simulink model "ysw_PID2"  (Simulink 8.3)
settings: Solver=ode45  StartTime=0.0  StopTime=10  RelTol=1e-3
values from neighbouring files (symbols this model uses):
  A = [  0 ,     1,                 0                 0 ... (first row only)    [ysw_PID.m]
  B = [0;  (I+m*l^2)/((M+m)*I+M*m*l^2);  0;  m*l/(((M+m)*I+M*m*l^2))]    [ysw_PID.m]
  C = [1 0 0 0;0 1 0 0;0 0 1 0;0 0 0 1]    [ysw_PID.m]
  D = [0;0;0;0]    [ysw_PID.m]
  K = place(A,B,p)    [ysw_PID.m]
libraries: simulink x1
settings Model: Creator=ii  LastModifiedBy=ii
settings SolverCC: ZeroCrossAlgorithm=Adaptive
settings DataIOCC: SignalLoggingSaveFormat=Dataset
settings DebuggingCC: StateNameClashWarn=none
settings GRTTargetCC: CombineOutputUpdateFcns=on  GRTInterface=off

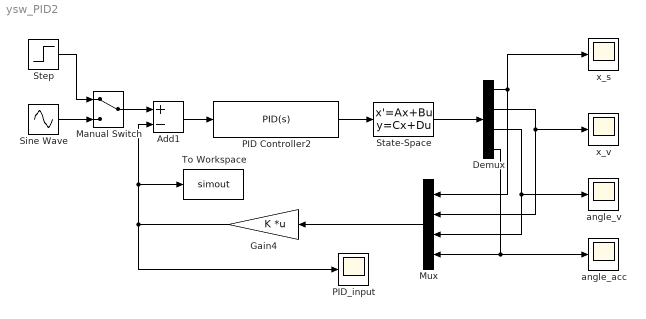
== system ysw_PID2 ==
  Add1 : Sum  Inputs=+-
  Demux : Demux
  Gain4 : Gain  Gain=K  Multiplication=Matrix(K*u)
  Manual Switch : ManualSwitch
  Mux : Mux
  PID Controller2 : simulink/Continuous/PID Controller  Controller=PID  TimeDomain=Continuous-time  SampleTime=1  IntegratorMethod=Forward Euler  FilterMethod=Forward Euler  Form=Parallel  P=5  I=0.001  D=1  N=100  InitialConditionSource=internal  InitialConditionForIntegrator=0  InitialConditionForFilter=0  ExternalReset=none  LimitOutput=off  UpperSaturationLimit=inf  LowerSaturationLimit=-inf  LinearizeAsGain=on  AntiWindupMode=none  Kb=1  TrackingMode=off  Kt=1  PParamMin=[]  PParamMax=[]  IParamMin=[]  IParamMax=[]  DParamMin=[]  DParamMax=[]  NParamMin=[]  NParamMax=[]  KbParamMin=[]  KbParamMax=[]  KtParamMin=[]  KtParamMax=[]  POutMin=[]  POutMax=[]  IOutMin=[]  IOutMax=[]  DOutMin=[]  DOutMax=[]  NOutMin=[]  NOutMax=[]  KbOutMin=[]  KbOutMax=[]  KtOutMin=[]  KtOutMax=[]  IntegratorOutMin=[]  IntegratorOutMax=[]  FilterOutMin=[]  FilterOutMax=[]  SumOutMin=[]  SumOutMax=[]  SumI1OutMin=[]  SumI1OutMax=[]  SumI2OutMin=[]  SumI2OutMax=[]  SumI3OutMin=[]  SumI3OutMax=[]  SumDOutMin=[]  SumDOutMax=[]  SaturationOutMin=[]  SaturationOutMax=[]  IntegratorContinuousStateAttributes=''  IntegratorStateMustResolveToSignalObject=off  IntegratorRTWStateStorageClass=Auto  FilterContinuousStateAttributes=''  FilterStateMustResolveToSignalObject=off  FilterRTWStateStorageClass=Auto
  PID_input : Scope
      settings: SaveName=ScopeData4
  Sine Wave : Sin  SampleTime=0
  State-Space : StateSpace  A=A  B=B  C=C  D=D  X0=0
  Step : Step  SampleTime=0
  To Workspace : ToWorkspace  VariableName=simout  SampleTime=-1
  angle_acc : Scope
      settings: SaveName=ScopeData3
  angle_v : Scope
      settings: SaveName=ScopeData2
  x_s : Scope
  x_v : Scope
  wires:
  Add1/1 -> PID Controller2/1
  PID Controller2/1 -> State-Space/1
  Gain4/1 -> To Workspace/1, Add1/2, PID_input/1
  State-Space/1 -> Demux/1
  Mux/1 -> Gain4/1
  Demux/1 -> x_s/1, Mux/1
  Demux/4 -> Mux/4, angle_acc/1
  Demux/3 -> Mux/3, angle_v/1
  Demux/2 -> x_v/1, Mux/2
  Step/1 -> Manual Switch/1
  Sine Wave/1 -> Manual Switch/2
  Manual Switch/1 -> Add1/1
